simulink model "observer_fb_sim"  (R2020a)
settings: Solver=VariableStepAuto  StartTime=0.0  StopTime=5  RelTol=1e-6
undefined symbols (not defined in the file): icd, K, L, sysd, T
settings Model: Creator=Jasper  LastModifiedBy=Jasper

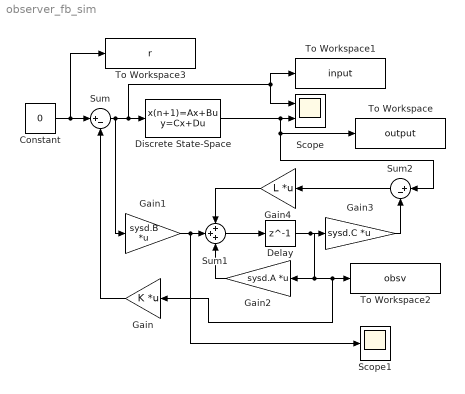
== system observer_fb_sim ==
  Constant : Constant  Value=0
  Delay : Delay  DelayLength=1  SampleTime=T
  Discrete State-Space : DiscreteStateSpace  A=sysd.A  B=sysd.B  C=sysd.C  D=sysd.D  InitialCondition=icd  SampleTime=-1
  Gain : Gain  Gain=K  Multiplication=Matrix(K*u)
  Gain1 : Gain  Gain=sysd.B  Multiplication=Matrix(K*u)
  Gain2 : Gain  Gain=sysd.A  Multiplication=Matrix(K*u)
  Gain3 : Gain  Gain=sysd.C  Multiplication=Matrix(K*u)
  Gain4 : Gain  Gain=L  Multiplication=Matrix(K*u)
  Scope : Scope  NumInputPorts=2
  Scope1 : Scope
  Sum : Sum  Inputs=|+-
  Sum1 : Sum  Inputs=+++
  Sum2 : Sum  Inputs=|+-
  To Workspace : ToWorkspace  VariableName=output  SaveFormat=Timeseries  SampleTime=-1
  To Workspace1 : ToWorkspace  VariableName=input  SaveFormat=Timeseries  SampleTime=-1
  To Workspace2 : ToWorkspace  VariableName=obsv  SaveFormat=Timeseries  SampleTime=-1
  To Workspace3 : ToWorkspace  VariableName=r  SaveFormat=Timeseries  SampleTime=-1
  wires:
  Discrete State-Space/1 -> To Workspace/1, Sum2/1, Scope/2
  Gain/1 -> Sum/2
  Sum/1 -> Discrete State-Space/1, Scope/1, To Workspace1/1, Gain1/1
  Constant/1 -> To Workspace3/1, Sum/1
  Sum1/1 -> Delay/1
  Delay/1 -> Gain2/1, Gain/1, To Workspace2/1, Gain3/1
  Gain3/1 -> Sum2/2
  Gain1/1 -> Scope1/1, Sum1/2
  Gain2/1 -> Sum1/3
  Sum2/1 -> Gain4/1
  Gain4/1 -> Sum1/1
